simulink model "BLOC_RA_TQ_to_F_BRAKE"  (R2016a)
settings: Solver=VariableStepAuto  StartTime=0.0  StopTime=10.0  RelTol=1e-3
undefined symbols (not defined in the file): hev_dt, pla_wheel_radius
settings Model: Creator=Florent  LastModifiedBy=Florent

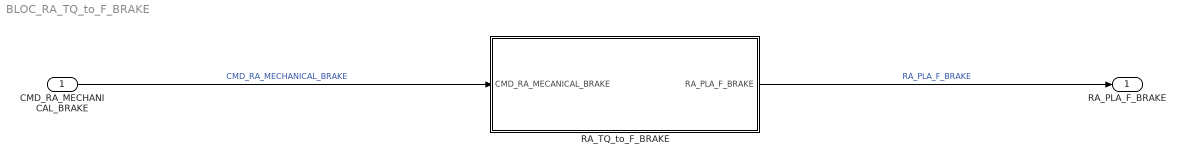
== system BLOC_RA_TQ_to_F_BRAKE ==
  CMD_RA_MECHANICAL_BRAKE : Inport
  RA_TQ_to_F_BRAKE : Subsystem  TreatAsAtomicUnit=on  SystemSampleTime=hev_dt
  RA_PLA_F_BRAKE : Outport
  wires:
  RA_TQ_to_F_BRAKE/1(RA_PLA_F_BRAKE) -> RA_PLA_F_BRAKE/1  "RA_PLA_F_BRAKE"
  CMD_RA_MECHANICAL_BRAKE/1 -> RA_TQ_to_F_BRAKE/1(CMD_RA_MECANICAL_BRAKE)  "CMD_RA_MECHANICAL_BRAKE"

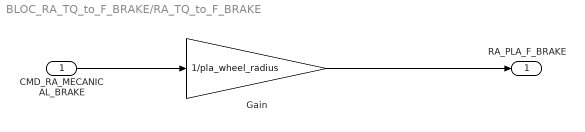
== system BLOC_RA_TQ_to_F_BRAKE/RA_TQ_to_F_BRAKE ==
  CMD_RA_MECANICAL_BRAKE : Inport
  Gain : Gain  Gain=1/pla_wheel_radius
  RA_PLA_F_BRAKE : Outport
  wires:
  CMD_RA_MECANICAL_BRAKE/1 -> Gain/1
  Gain/1 -> RA_PLA_F_BRAKE/1
